simulink model "MyPTControl_RTW"  (Simulink 8.7)
settings: Solver=ode1  SolverMode=SingleTasking  StartTime=0.0  StopTime=inf  FixedStep=0.001  RelTol=1e-3
PreLoadFcn:
  | vehicle = 'Car'; if ~length(which('cmcmd')), cmenv; end
  | MyPTControl_RTW_bus
InitFcn:
  | vehicle = 'Car'; if ~length(which('cmcmd')), cmenv; end
  | MyPTControl_RTW_bus
undefined symbols (not defined in the file or in its folder): EngineOut_Load, EngineOut_set_ISC, Ignition, ISGOut_Load, OperationState
libraries: simulink x11
Description:
  | CarMaker Plug-in Model Target
settings Model: Creator=ml  LastModifiedBy=IPG
settings DataIOCC: SignalLoggingSaveFormat=ModelDataLogs
settings OptimizationCC: ExpressionDepthLimit=2147483647
settings DebuggingCC: FcnCallInpInsideContextMsg=EnableAllAsWarning  StateNameClashWarn=warning
settings HardwareCC: TargetHWDeviceType=32-bit Generic  ProdEqTarget=off
settings RTWCC: SystemTargetFile=CarMaker.tlc  TemplateMakefile=CarMaker_unix-win64.tmf  Description=CarMaker Plug-in Model Target
settings CodeAppCC: MaxIdLength=127
settings STFCustomTargetCC: ModelReferenceCompliant=off  GeneratePreprocessorConditionals=Disable all  MultiInstanceERTCode=on  CodeInterfacePackaging=Reusable function  CPPClassGenCompliant=on  GRTInterface=off  GenerateAllocFcn=on  SystemTargetFile=CarMaker.tlc
settings GRTTargetCC: ModelReferenceCompliant=off  ParMdlRefBuildCompliant=off  CompOptLevelCompliant=off  ConcurrentExecutionCompliant=off  CombineOutputUpdateFcns=off  MatFileLogging=off  MultiInstanceERTCode=on  CodeInterfacePackaging=Reusable function  GenerateAllocFcn=on  UseToolchainInfoCompliant=off
settings CustomProperty: DataType=string  Value=..
settings EnumStrPairs: String=Car

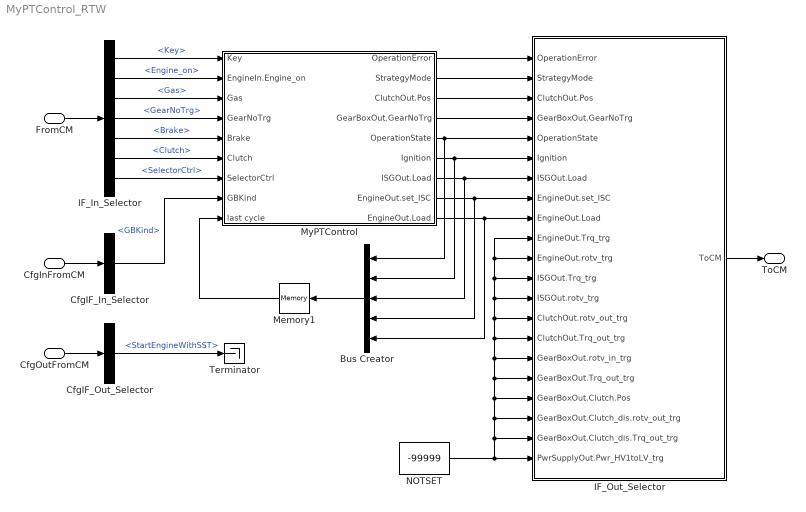
== system MyPTControl_RTW ==
  FromCM : Inport  OutDataTypeStr=Bus: cmPTControlIn
  CfgInFromCM : Inport  Port=2  OutDataTypeStr=Bus: cmPTControlCfgIn
  CfgOutFromCM : Inport  Port=3  OutDataTypeStr=Bus: cmPTControlCfgOut
  Bus Creator : BusCreator  Inputs=5
  CfgIF_In_Selector : BusSelector  OutputSignals=GearBox.GBKind
  CfgIF_Out_Selector : BusSelector  OutputSignals=StartEngineWithSST
  IF_In_Selector : BusSelector  OutputSignals=Key,EngineIn.Engine_on,Gas,GearNoTrg,Brake,Clutch,SelectorCtrl
  IF_Out_Selector : Subsystem  mask(Signal Selection){}
      mask help: Signal Selection Block
      settings: OpenFcn=cmSignalSelect('SignalSelection_CB',gcb)
  Memory1 : Memory
  MyPTControl : Subsystem
  NOTSET : Constant  Value=-99999
  Terminator : Terminator
  ToCM : Outport  OutDataTypeStr=Bus: cmPTControlOut
  wires:
  FromCM/1 -> IF_In_Selector/1
  IF_Out_Selector/1(ToCM) -> ToCM/1
  CfgInFromCM/1 -> CfgIF_In_Selector/1
  CfgOutFromCM/1 -> CfgIF_Out_Selector/1
  Bus Creator/1 -> Memory1/1
  Memory1/1 -> MyPTControl/9(last cycle)
  MyPTControl/5(OperationState) -> Bus Creator/1, IF_Out_Selector/5(OperationState)
  MyPTControl/6(Ignition) -> Bus Creator/2, IF_Out_Selector/6(Ignition)
  MyPTControl/7(ISGOut.Load) -> Bus Creator/3, IF_Out_Selector/7(ISGOut.Load)
  MyPTControl/8(EngineOut.set_ISC) -> Bus Creator/4, IF_Out_Selector/8(EngineOut.set_ISC)
  MyPTControl/9(EngineOut.Load) -> Bus Creator/5, IF_Out_Selector/9(EngineOut.Load)
  MyPTControl/1(OperationError) -> IF_Out_Selector/1(OperationError)
  MyPTControl/2(StrategyMode) -> IF_Out_Selector/2(StrategyMode)
  MyPTControl/3(ClutchOut.Pos) -> IF_Out_Selector/3(ClutchOut.Pos)
  MyPTControl/4(GearBoxOut.GearNoTrg) -> IF_Out_Selector/4(GearBoxOut.GearNoTrg)
  IF_In_Selector/1 -> MyPTControl/1(Key)  "<Key>"
  IF_In_Selector/2 -> MyPTControl/2(EngineIn.Engine_on)  "<Engine_on>"
  IF_In_Selector/3 -> MyPTControl/3(Gas)  "<Gas>"
  IF_In_Selector/4 -> MyPTControl/4(GearNoTrg)  "<GearNoTrg>"
  IF_In_Selector/5 -> MyPTControl/5(Brake)  "<Brake>"
  IF_In_Selector/6 -> MyPTControl/6(Clutch)  "<Clutch>"
  IF_In_Selector/7 -> MyPTControl/7(SelectorCtrl)  "<SelectorCtrl>"
  CfgIF_In_Selector/1 -> MyPTControl/8(GBKind)  "<GBKind>"
  CfgIF_Out_Selector/1 -> Terminator/1  "<StartEngineWithSST>"
  NOTSET/1 -> IF_Out_Selector/21(PwrSupplyOut.Pwr_HV1toLV_trg), IF_Out_Selector/10(EngineOut.Trq_trg), IF_Out_Selector/11(EngineOut.rotv_trg), IF_Out_Selector/12(ISGOut.Trq_trg), IF_Out_Selector/13(ISGOut.rotv_trg), IF_Out_Selector/14(ClutchOut.rotv_out_trg), IF_Out_Selector/15(ClutchOut.Trq_out_trg), IF_Out_Selector/16(GearBoxOut.rotv_in_trg), IF_Out_Selector/17(GearBoxOut.Trq_out_trg), IF_Out_Selector/18(GearBoxOut.Clutch.Pos), IF_Out_Selector/19(GearBoxOut.Clutch_dis.rotv_out_trg), IF_Out_Selector/20(GearBoxOut.Clutch_dis.Trq_out_trg)

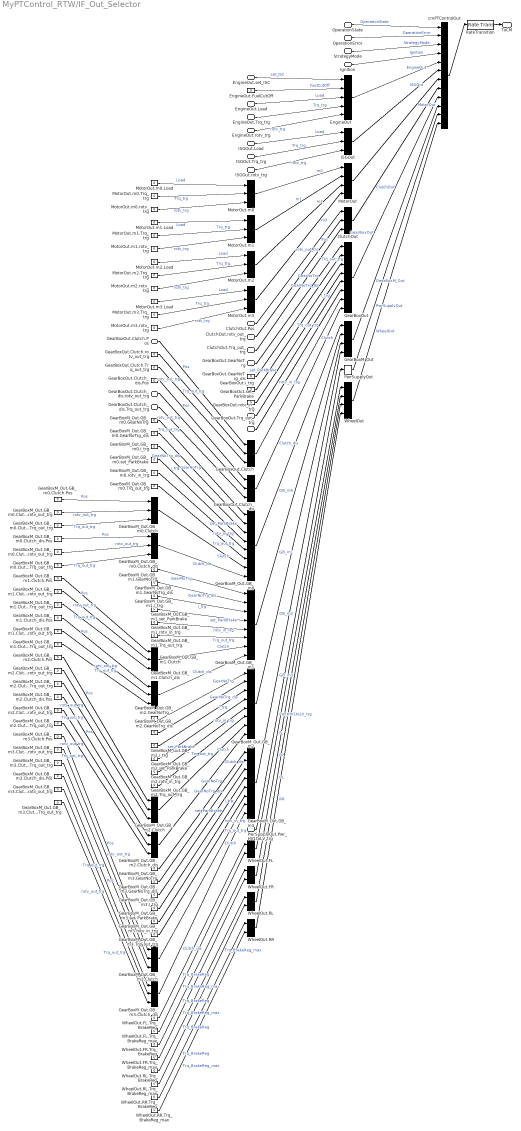
== system MyPTControl_RTW/IF_Out_Selector ==
  OperationError : Inport
  StrategyMode : Inport  Port=2
  ClutchOut.Pos : Inport  Port=3
  GearBoxOut.GearNoTrg : Inport  Port=4
  OperationState : Inport  Port=5
  Ignition : Inport  Port=6
  ISGOut.Load : Inport  Port=7
  EngineOut.set_ISC : Inport  Port=8
  EngineOut.Load : Inport  Port=9
  EngineOut.Trq_trg : Inport  Port=10
  EngineOut.rotv_trg : Inport  Port=11
  ISGOut.Trq_trg : Inport  Port=12
  ISGOut.rotv_trg : Inport  Port=13
  ClutchOut.rotv_out_trg : Inport  Port=14
  ClutchOut.Trq_out_trg : Inport  Port=15
  GearBoxOut.rotv_in_trg : Inport  Port=16
  GearBoxOut.Trq_out_trg : Inport  Port=17
  GearBoxOut.Clutch.Pos : Inport  Port=18
  GearBoxOut.Clutch_dis.rotv_out_trg : Inport  Port=19
  GearBoxOut.Clutch_dis.Trq_out_trg : Inport  Port=20
  PwrSupplyOut.Pwr_HV1toLV_trg : Inport  Port=21
  ClutchOut : BusCreator  Inputs=3
  EngineOut : BusCreator  Inputs=5
  EngineOut.FuelCutOff : Constant  Value=0
  GearBoxM_Out : BusCreator  Inputs=4
  GearBoxM_Out.GB_m{0..3} (4 alike) : BusCreator  Inputs=8
  GearBoxM_Out.GB_m0.Clutch : BusCreator  Inputs=3
  GearBoxM_Out.GB_m0.Clutch.Pos : Constant  Value=0
  GearBoxM_Out.GB_m0.Clutch.Trq_out_trg : Constant  Value=0
  GearBoxM_Out.GB_m0.Clutch.rotv_out_trg : Constant  Value=0
  GearBoxM_Out.GB_m0.Clutch_dis : BusCreator  Inputs=3
  GearBoxM_Out.GB_m0.Clutch_dis.Pos : Constant  Value=0
  GearBoxM_Out.GB_m0.Clutch_dis.Trq_out_trg : Constant  Value=0
  GearBoxM_Out.GB_m0.Clutch_dis.rotv_out_trg : Constant  Value=0
  GearBoxM_Out.GB_m0.GearNoTrg : Constant  Value=0
  GearBoxM_Out.GB_m0.GearNoTrg_dis : Constant  Value=0
  GearBoxM_Out.GB_m0.Trq_out_trg : Constant  Value=0
  GearBoxM_Out.GB_m0.i_trg : Constant  Value=0
  GearBoxM_Out.GB_m0.rotv_in_trg : Constant  Value=0
  GearBoxM_Out.GB_m0.set_ParkBrake : Constant  Value=0
  GearBoxM_Out.GB_m1.Clutch : BusCreator  Inputs=3
  GearBoxM_Out.GB_m1.Clutch.Pos : Constant  Value=0
  GearBoxM_Out.GB_m1.Clutch.Trq_out_trg : Constant  Value=0
  GearBoxM_Out.GB_m1.Clutch.rotv_out_trg : Constant  Value=0
  GearBoxM_Out.GB_m1.Clutch_dis : BusCreator  Inputs=3
  GearBoxM_Out.GB_m1.Clutch_dis.Pos : Constant  Value=0
  GearBoxM_Out.GB_m1.Clutch_dis.Trq_out_trg : Constant  Value=0
  GearBoxM_Out.GB_m1.Clutch_dis.rotv_out_trg : Constant  Value=0
  GearBoxM_Out.GB_m1.GearNoTrg : Constant  Value=0
  GearBoxM_Out.GB_m1.GearNoTrg_dis : Constant  Value=0
  GearBoxM_Out.GB_m1.Trq_out_trg : Constant  Value=0
  GearBoxM_Out.GB_m1.i_trg : Constant  Value=0
  GearBoxM_Out.GB_m1.rotv_in_trg : Constant  Value=0
  GearBoxM_Out.GB_m1.set_ParkBrake : Constant  Value=0
  GearBoxM_Out.GB_m2.Clutch : BusCreator  Inputs=3
  GearBoxM_Out.GB_m2.Clutch.Pos : Constant  Value=0
  GearBoxM_Out.GB_m2.Clutch.Trq_out_trg : Constant  Value=0
  GearBoxM_Out.GB_m2.Clutch.rotv_out_trg : Constant  Value=0
  GearBoxM_Out.GB_m2.Clutch_dis : BusCreator  Inputs=3
  GearBoxM_Out.GB_m2.Clutch_dis.Pos : Constant  Value=0
  GearBoxM_Out.GB_m2.Clutch_dis.Trq_out_trg : Constant  Value=0
  GearBoxM_Out.GB_m2.Clutch_dis.rotv_out_trg : Constant  Value=0
  GearBoxM_Out.GB_m2.GearNoTrg : Constant  Value=0
  GearBoxM_Out.GB_m2.GearNoTrg_dis : Constant  Value=0
  GearBoxM_Out.GB_m2.Trq_out_trg : Constant  Value=0
  GearBoxM_Out.GB_m2.i_trg : Constant  Value=0
  GearBoxM_Out.GB_m2.rotv_in_trg : Constant  Value=0
  GearBoxM_Out.GB_m2.set_ParkBrake : Constant  Value=0
  GearBoxM_Out.GB_m3.Clutch : BusCreator  Inputs=3
  GearBoxM_Out.GB_m3.Clutch.Pos : Constant  Value=0
  GearBoxM_Out.GB_m3.Clutch.Trq_out_trg : Constant  Value=0
  GearBoxM_Out.GB_m3.Clutch.rotv_out_trg : Constant  Value=0
  GearBoxM_Out.GB_m3.Clutch_dis : BusCreator  Inputs=3
  GearBoxM_Out.GB_m3.Clutch_dis.Pos : Constant  Value=0
  GearBoxM_Out.GB_m3.Clutch_dis.Trq_out_trg : Constant  Value=0
  GearBoxM_Out.GB_m3.Clutch_dis.rotv_out_trg : Constant  Value=0
  GearBoxM_Out.GB_m3.GearNoTrg : Constant  Value=0
  GearBoxM_Out.GB_m3.GearNoTrg_dis : Constant  Value=0
  GearBoxM_Out.GB_m3.Trq_out_trg : Constant  Value=0
  GearBoxM_Out.GB_m3.i_trg : Constant  Value=0
  GearBoxM_Out.GB_m3.rotv_in_trg : Constant  Value=0
  GearBoxM_Out.GB_m3.set_ParkBrake : Constant  Value=0
  GearBoxOut : BusCreator  Inputs=8
  GearBoxOut.Clutch : BusCreator  Inputs=3
  GearBoxOut.Clutch.Trq_out_trg : Constant  Value=0
  GearBoxOut.Clutch.rotv_out_trg : Constant  Value=0
  GearBoxOut.Clutch_dis : BusCreator  Inputs=3
  GearBoxOut.Clutch_dis.Pos : Constant  Value=0
  GearBoxOut.GearNoTrg_dis : Constant  Value=0
  GearBoxOut.i_trg : Constant  Value=0
  GearBoxOut.set_ParkBrake : Constant  Value=0
  ISGOut : BusCreator  Inputs=3
  MotorOut : BusCreator  Inputs=4
  MotorOut.m{0..3} (4 alike) : BusCreator  Inputs=3
  MotorOut.m0.Load : Constant  Value=0
  MotorOut.m0.Trq_trg : Constant  Value=0
  MotorOut.m0.rotv_trg : Constant  Value=0
  MotorOut.m1.Load : Constant  Value=0
  MotorOut.m1.Trq_trg : Constant  Value=0
  MotorOut.m1.rotv_trg : Constant  Value=0
  MotorOut.m2.Load : Constant  Value=0
  MotorOut.m2.Trq_trg : Constant  Value=0
  MotorOut.m2.rotv_trg : Constant  Value=0
  MotorOut.m3.Load : Constant  Value=0
  MotorOut.m3.Trq_trg : Constant  Value=0
  MotorOut.m3.rotv_trg : Constant  Value=0
  PwrSupplyOut : BusCreator  Inputs=1
  RateTransition : RateTransition  OutPortSampleTime=str2num(get_param(bdroot,'FixedStep'))
  WheelOut : BusCreator  Inputs=4
  WheelOut.FL : BusCreator  Inputs=2
  WheelOut.FL.Trq_BrakeReg : Constant  Value=0
  WheelOut.FL.Trq_BrakeReg_max : Constant  Value=0
  WheelOut.FR : BusCreator  Inputs=2
  WheelOut.FR.Trq_BrakeReg : Constant  Value=0
  WheelOut.FR.Trq_BrakeReg_max : Constant  Value=0
  WheelOut.RL : BusCreator  Inputs=2
  WheelOut.RL.Trq_BrakeReg : Constant  Value=0
  WheelOut.RL.Trq_BrakeReg_max : Constant  Value=0
  WheelOut.RR : BusCreator  Inputs=2
  WheelOut.RR.Trq_BrakeReg : Constant  Value=0
  WheelOut.RR.Trq_BrakeReg_max : Constant  Value=0
  cmPTControlOut : BusCreator  Inputs=12
  ToCM : Outport
  wires:
  RateTransition/1 -> ToCM/1
  cmPTControlOut/1 -> RateTransition/1
  EngineOut/1 -> cmPTControlOut/5  "EngineOut"
  EngineOut.FuelCutOff/1 -> EngineOut/2  "FuelCutOff"
  ISGOut/1 -> cmPTControlOut/6  "ISGOut"
  MotorOut/1 -> cmPTControlOut/7  "MotorOut"
  MotorOut.m0/1 -> MotorOut/1  "m0"
  MotorOut.m0.Load/1 -> MotorOut.m0/1  "Load"
  MotorOut.m0.Trq_trg/1 -> MotorOut.m0/2  "Trq_trg"
  MotorOut.m0.rotv_trg/1 -> MotorOut.m0/3  "rotv_trg"
  MotorOut.m1/1 -> MotorOut/2  "m1"
  MotorOut.m1.Load/1 -> MotorOut.m1/1  "Load"
  MotorOut.m1.Trq_trg/1 -> MotorOut.m1/2  "Trq_trg"
  MotorOut.m1.rotv_trg/1 -> MotorOut.m1/3  "rotv_trg"
  MotorOut.m2/1 -> MotorOut/3  "m2"
  MotorOut.m2.Load/1 -> MotorOut.m2/1  "Load"
  MotorOut.m2.Trq_trg/1 -> MotorOut.m2/2  "Trq_trg"
  MotorOut.m2.rotv_trg/1 -> MotorOut.m2/3  "rotv_trg"
  MotorOut.m3/1 -> MotorOut/4  "m3"
  MotorOut.m3.Load/1 -> MotorOut.m3/1  "Load"
  MotorOut.m3.Trq_trg/1 -> MotorOut.m3/2  "Trq_trg"
  MotorOut.m3.rotv_trg/1 -> MotorOut.m3/3  "rotv_trg"
  ClutchOut/1 -> cmPTControlOut/8  "ClutchOut"
  GearBoxOut/1 -> cmPTControlOut/9  "GearBoxOut"
  GearBoxOut.GearNoTrg_dis/1 -> GearBoxOut/2  "GearNoTrg_dis"
  GearBoxOut.i_trg/1 -> GearBoxOut/3  "i_trg"
  GearBoxOut.set_ParkBrake/1 -> GearBoxOut/4  "set_ParkBrake"
  GearBoxOut.Clutch/1 -> GearBoxOut/7  "Clutch"
  GearBoxOut.Clutch.rotv_out_trg/1 -> GearBoxOut.Clutch/2  "rotv_out_trg"
  GearBoxOut.Clutch.Trq_out_trg/1 -> GearBoxOut.Clutch/3  "Trq_out_trg"
  GearBoxOut.Clutch_dis/1 -> GearBoxOut/8  "Clutch_dis"
  GearBoxOut.Clutch_dis.Pos/1 -> GearBoxOut.Clutch_dis/1  "Pos"
  GearBoxM_Out/1 -> cmPTControlOut/10  "GearBoxM_Out"
  GearBoxM_Out.GB_m0/1 -> GearBoxM_Out/1  "GB_m0"
  GearBoxM_Out.GB_m0.GearNoTrg/1 -> GearBoxM_Out.GB_m0/1  "GearNoTrg"
  GearBoxM_Out.GB_m0.GearNoTrg_dis/1 -> GearBoxM_Out.GB_m0/2  "GearNoTrg_dis"
  GearBoxM_Out.GB_m0.i_trg/1 -> GearBoxM_Out.GB_m0/3  "i_trg"
  GearBoxM_Out.GB_m0.set_ParkBrake/1 -> GearBoxM_Out.GB_m0/4  "set_ParkBrake"
  GearBoxM_Out.GB_m0.rotv_in_trg/1 -> GearBoxM_Out.GB_m0/5  "rotv_in_trg"
  GearBoxM_Out.GB_m0.Trq_out_trg/1 -> GearBoxM_Out.GB_m0/6  "Trq_out_trg"
  GearBoxM_Out.GB_m0.Clutch/1 -> GearBoxM_Out.GB_m0/7  "Clutch"
  GearBoxM_Out.GB_m0.Clutch.Pos/1 -> GearBoxM_Out.GB_m0.Clutch/1  "Pos"
  GearBoxM_Out.GB_m0.Clutch.rotv_out_trg/1 -> GearBoxM_Out.GB_m0.Clutch/2  "rotv_out_trg"
  GearBoxM_Out.GB_m0.Clutch.Trq_out_trg/1 -> GearBoxM_Out.GB_m0.Clutch/3  "Trq_out_trg"
  GearBoxM_Out.GB_m0.Clutch_dis/1 -> GearBoxM_Out.GB_m0/8  "Clutch_dis"
  GearBoxM_Out.GB_m0.Clutch_dis.Pos/1 -> GearBoxM_Out.GB_m0.Clutch_dis/1  "Pos"
  GearBoxM_Out.GB_m0.Clutch_dis.rotv_out_trg/1 -> GearBoxM_Out.GB_m0.Clutch_dis/2  "rotv_out_trg"
  GearBoxM_Out.GB_m0.Clutch_dis.Trq_out_trg/1 -> GearBoxM_Out.GB_m0.Clutch_dis/3  "Trq_out_trg"
  GearBoxM_Out.GB_m1/1 -> GearBoxM_Out/2  "GB_m1"
  GearBoxM_Out.GB_m1.GearNoTrg/1 -> GearBoxM_Out.GB_m1/1  "GearNoTrg"
  GearBoxM_Out.GB_m1.GearNoTrg_dis/1 -> GearBoxM_Out.GB_m1/2  "GearNoTrg_dis"
  GearBoxM_Out.GB_m1.i_trg/1 -> GearBoxM_Out.GB_m1/3  "i_trg"
  GearBoxM_Out.GB_m1.set_ParkBrake/1 -> GearBoxM_Out.GB_m1/4  "set_ParkBrake"
  GearBoxM_Out.GB_m1.rotv_in_trg/1 -> GearBoxM_Out.GB_m1/5  "rotv_in_trg"
  GearBoxM_Out.GB_m1.Trq_out_trg/1 -> GearBoxM_Out.GB_m1/6  "Trq_out_trg"
  GearBoxM_Out.GB_m1.Clutch/1 -> GearBoxM_Out.GB_m1/7  "Clutch"
  GearBoxM_Out.GB_m1.Clutch.Pos/1 -> GearBoxM_Out.GB_m1.Clutch/1  "Pos"
  GearBoxM_Out.GB_m1.Clutch.rotv_out_trg/1 -> GearBoxM_Out.GB_m1.Clutch/2  "rotv_out_trg"
  GearBoxM_Out.GB_m1.Clutch.Trq_out_trg/1 -> GearBoxM_Out.GB_m1.Clutch/3  "Trq_out_trg"
  GearBoxM_Out.GB_m1.Clutch_dis/1 -> GearBoxM_Out.GB_m1/8  "Clutch_dis"
  GearBoxM_Out.GB_m1.Clutch_dis.Pos/1 -> GearBoxM_Out.GB_m1.Clutch_dis/1  "Pos"
  GearBoxM_Out.GB_m1.Clutch_dis.rotv_out_trg/1 -> GearBoxM_Out.GB_m1.Clutch_dis/2  "rotv_out_trg"
  GearBoxM_Out.GB_m1.Clutch_dis.Trq_out_trg/1 -> GearBoxM_Out.GB_m1.Clutch_dis/3  "Trq_out_trg"
  GearBoxM_Out.GB_m2/1 -> GearBoxM_Out/3  "GB_m2"
  GearBoxM_Out.GB_m2.GearNoTrg/1 -> GearBoxM_Out.GB_m2/1  "GearNoTrg"
  GearBoxM_Out.GB_m2.GearNoTrg_dis/1 -> GearBoxM_Out.GB_m2/2  "GearNoTrg_dis"
  GearBoxM_Out.GB_m2.i_trg/1 -> GearBoxM_Out.GB_m2/3  "i_trg"
  GearBoxM_Out.GB_m2.set_ParkBrake/1 -> GearBoxM_Out.GB_m2/4  "set_ParkBrake"
  GearBoxM_Out.GB_m2.rotv_in_trg/1 -> GearBoxM_Out.GB_m2/5  "rotv_in_trg"
  GearBoxM_Out.GB_m2.Trq_out_trg/1 -> GearBoxM_Out.GB_m2/6  "Trq_out_trg"
  GearBoxM_Out.GB_m2.Clutch/1 -> GearBoxM_Out.GB_m2/7  "Clutch"
  GearBoxM_Out.GB_m2.Clutch.Pos/1 -> GearBoxM_Out.GB_m2.Clutch/1  "Pos"
  GearBoxM_Out.GB_m2.Clutch.rotv_out_trg/1 -> GearBoxM_Out.GB_m2.Clutch/2  "rotv_out_trg"
  GearBoxM_Out.GB_m2.Clutch.Trq_out_trg/1 -> GearBoxM_Out.GB_m2.Clutch/3  "Trq_out_trg"
  GearBoxM_Out.GB_m2.Clutch_dis/1 -> GearBoxM_Out.GB_m2/8  "Clutch_dis"
  GearBoxM_Out.GB_m2.Clutch_dis.Pos/1 -> GearBoxM_Out.GB_m2.Clutch_dis/1  "Pos"
  GearBoxM_Out.GB_m2.Clutch_dis.rotv_out_trg/1 -> GearBoxM_Out.GB_m2.Clutch_dis/2  "rotv_out_trg"
  GearBoxM_Out.GB_m2.Clutch_dis.Trq_out_trg/1 -> GearBoxM_Out.GB_m2.Clutch_dis/3  "Trq_out_trg"
  GearBoxM_Out.GB_m3/1 -> GearBoxM_Out/4  "GB_m3"
  GearBoxM_Out.GB_m3.GearNoTrg/1 -> GearBoxM_Out.GB_m3/1  "GearNoTrg"
  GearBoxM_Out.GB_m3.GearNoTrg_dis/1 -> GearBoxM_Out.GB_m3/2  "GearNoTrg_dis"
  GearBoxM_Out.GB_m3.i_trg/1 -> GearBoxM_Out.GB_m3/3  "i_trg"
  GearBoxM_Out.GB_m3.set_ParkBrake/1 -> GearBoxM_Out.GB_m3/4  "set_ParkBrake"
  GearBoxM_Out.GB_m3.rotv_in_trg/1 -> GearBoxM_Out.GB_m3/5  "rotv_in_trg"
  GearBoxM_Out.GB_m3.Trq_out_trg/1 -> GearBoxM_Out.GB_m3/6  "Trq_out_trg"
  GearBoxM_Out.GB_m3.Clutch/1 -> GearBoxM_Out.GB_m3/7  "Clutch"
  GearBoxM_Out.GB_m3.Clutch.Pos/1 -> GearBoxM_Out.GB_m3.Clutch/1  "Pos"
  GearBoxM_Out.GB_m3.Clutch.rotv_out_trg/1 -> GearBoxM_Out.GB_m3.Clutch/2  "rotv_out_trg"
  GearBoxM_Out.GB_m3.Clutch.Trq_out_trg/1 -> GearBoxM_Out.GB_m3.Clutch/3  "Trq_out_trg"
  GearBoxM_Out.GB_m3.Clutch_dis/1 -> GearBoxM_Out.GB_m3/8  "Clutch_dis"
  GearBoxM_Out.GB_m3.Clutch_dis.Pos/1 -> GearBoxM_Out.GB_m3.Clutch_dis/1  "Pos"
  GearBoxM_Out.GB_m3.Clutch_dis.rotv_out_trg/1 -> GearBoxM_Out.GB_m3.Clutch_dis/2  "rotv_out_trg"
  GearBoxM_Out.GB_m3.Clutch_dis.Trq_out_trg/1 -> GearBoxM_Out.GB_m3.Clutch_dis/3  "Trq_out_trg"
  PwrSupplyOut/1 -> cmPTControlOut/11  "PwrSupplyOut"
  WheelOut/1 -> cmPTControlOut/12  "WheelOut"
  WheelOut.FL/1 -> WheelOut/1  "FL"
  WheelOut.FL.Trq_BrakeReg/1 -> WheelOut.FL/1  "Trq_BrakeReg"
  WheelOut.FL.Trq_BrakeReg_max/1 -> WheelOut.FL/2  "Trq_BrakeReg_max"
  WheelOut.FR/1 -> WheelOut/2  "FR"
  WheelOut.FR.Trq_BrakeReg/1 -> WheelOut.FR/1  "Trq_BrakeReg"
  WheelOut.FR.Trq_BrakeReg_max/1 -> WheelOut.FR/2  "Trq_BrakeReg_max"
  WheelOut.RL/1 -> WheelOut/3  "RL"
  WheelOut.RL.Trq_BrakeReg/1 -> WheelOut.RL/1  "Trq_BrakeReg"
  WheelOut.RL.Trq_BrakeReg_max/1 -> WheelOut.RL/2  "Trq_BrakeReg_max"
  WheelOut.RR/1 -> WheelOut/4  "RR"
  WheelOut.RR.Trq_BrakeReg/1 -> WheelOut.RR/1  "Trq_BrakeReg"
  WheelOut.RR.Trq_BrakeReg_max/1 -> WheelOut.RR/2  "Trq_BrakeReg_max"
  OperationError/1 -> cmPTControlOut/2  "OperationError"
  StrategyMode/1 -> cmPTControlOut/3  "StrategyMode"
  ClutchOut.Pos/1 -> ClutchOut/1  "Pos"
  GearBoxOut.GearNoTrg/1 -> GearBoxOut/1  "GearNoTrg"
  OperationState/1 -> cmPTControlOut/1  "OperationState"
  Ignition/1 -> cmPTControlOut/4  "Ignition"
  ISGOut.Load/1 -> ISGOut/1  "Load"
  EngineOut.set_ISC/1 -> EngineOut/1  "set_ISC"
  EngineOut.Load/1 -> EngineOut/3  "Load"
  EngineOut.Trq_trg/1 -> EngineOut/4  "Trq_trg"
  EngineOut.rotv_trg/1 -> EngineOut/5  "rotv_trg"
  ISGOut.Trq_trg/1 -> ISGOut/2  "Trq_trg"
  ISGOut.rotv_trg/1 -> ISGOut/3  "rotv_trg"
  ClutchOut.rotv_out_trg/1 -> ClutchOut/2  "rotv_out_trg"
  ClutchOut.Trq_out_trg/1 -> ClutchOut/3  "Trq_out_trg"
  GearBoxOut.rotv_in_trg/1 -> GearBoxOut/5  "rotv_in_trg"
  GearBoxOut.Trq_out_trg/1 -> GearBoxOut/6  "Trq_out_trg"
  GearBoxOut.Clutch.Pos/1 -> GearBoxOut.Clutch/1  "Pos"
  GearBoxOut.Clutch_dis.rotv_out_trg/1 -> GearBoxOut.Clutch_dis/2  "rotv_out_trg"
  GearBoxOut.Clutch_dis.Trq_out_trg/1 -> GearBoxOut.Clutch_dis/3  "Trq_out_trg"
  PwrSupplyOut.Pwr_HV1toLV_trg/1 -> PwrSupplyOut/1  "Pwr_HV1toLV_trg"

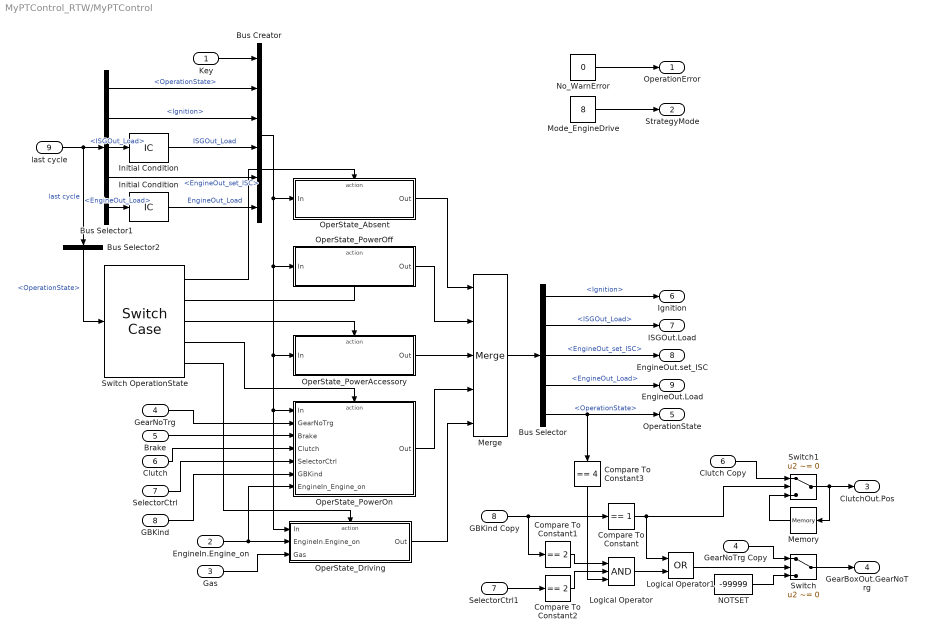
== system MyPTControl_RTW/MyPTControl ==
  Key : Inport
  EngineIn.Engine_on : Inport  Port=2
  Gas : Inport  Port=3
  GearNoTrg : Inport  Port=4
  Brake : Inport  Port=5
  Clutch : Inport  Port=6
  SelectorCtrl : Inport  Port=7
  GBKind : Inport  Port=8
  last cycle : Inport  Port=9
  Bus Creator : BusCreator  Inputs=6
  Bus Selector : BusSelector  OutputSignals=Ignition,ISGOut_Load,EngineOut_set_ISC,EngineOut_Load,OperationState
  Bus Selector1 : BusSelector  OutputSignals=OperationState,Ignition,ISGOut_Load,EngineOut_set_ISC,EngineOut_Load
  Bus Selector2 : BusSelector  OutputSignals=OperationState
  Clutch Copy : InportShadow  Port=6
  Compare To Constant : simulink/Logic and Bit Operations/Compare To Constant  relop===  const=1  OutDataTypeStr=uint8  ZeroCross=off
  Compare To Constant1 : simulink/Logic and Bit Operations/Compare To Constant  relop===  const=2  OutDataTypeStr=uint8  ZeroCross=off
  Compare To Constant2 : simulink/Logic and Bit Operations/Compare To Constant  relop===  const=2  OutDataTypeStr=uint8  ZeroCross=off
  Compare To Constant3 : simulink/Logic and Bit Operations/Compare To Constant  relop===  const=4  OutDataTypeStr=uint8  ZeroCross=off
  GBKind Copy : InportShadow  Port=8
  GearNoTrg Copy : InportShadow  Port=4
  Initial Condition : InitialCondition  Value=0
  "Initial Condition " : InitialCondition  Value=0
  Logical Operator : Logic  Inputs=3  AllPortsSameDT=off  OutDataTypeStr=boolean
  Logical Operator1 : Logic  Operator=OR  AllPortsSameDT=off  OutDataTypeStr=boolean
  Memory : Memory
  Merge : Merge  Inputs=5
  Mode_EngineDrive : Constant  Value=8
  NOTSET : Constant  Value=-99999
  No_WarnError : Constant  Value=0
  OperState_Absent : Subsystem  TreatAsAtomicUnit=on
  OperState_Driving : Subsystem  TreatAsAtomicUnit=on
  OperState_PowerAccessory : Subsystem  TreatAsAtomicUnit=on
  OperState_PowerOff : Subsystem  TreatAsAtomicUnit=on
  OperState_PowerOn : Subsystem  TreatAsAtomicUnit=on
  SelectorCtrl1 : InportShadow  Port=7
  Switch : Switch  Criteria=u2 ~= 0
  Switch OperationState : SwitchCase  CaseConditions={0 1 2 3}
  Switch1 : Switch  Criteria=u2 ~= 0
  OperationError : Outport
  StrategyMode : Outport  Port=2
  ClutchOut.Pos : Outport  Port=3
  GearBoxOut.GearNoTrg : Outport  Port=4
  OperationState : Outport  Port=5
  Ignition : Outport  Port=6
  ISGOut.Load : Outport  Port=7
  EngineOut.set_ISC : Outport  Port=8
  EngineOut.Load : Outport  Port=9
  wires:
  Compare To Constant3/1 -> Logical Operator/3
  GBKind Copy/1 -> Compare To Constant1/1, Compare To Constant/1
  SelectorCtrl1/1 -> Compare To Constant2/1
  OperState_Absent/1(Out) -> Merge/1
  Initial Condition/1 -> Bus Creator/4  "ISGOut_Load"
  "Initial Condition "/1 -> Bus Creator/6  "EngineOut_Load"
  Memory/1 -> Switch1/3
  Clutch Copy/1 -> Switch1/1
  Switch1/1 -> Memory/1, ClutchOut.Pos/1
  Switch/1 -> GearBoxOut.GearNoTrg/1
  GearNoTrg Copy/1 -> Switch/1
  NOTSET/1 -> Switch/3
  Logical Operator1/1 -> Switch/2
  Compare To Constant/1 -> Switch1/2, Logical Operator1/1
  Logical Operator/1 -> Logical Operator1/2
  Compare To Constant2/1 -> Logical Operator/2
  Compare To Constant1/1 -> Logical Operator/1
  Merge/1 -> Bus Selector/1
  OperState_Driving/1(Out) -> Merge/5
  OperState_PowerOn/1(Out) -> Merge/4
  OperState_PowerAccessory/1(Out) -> Merge/3
  OperState_PowerOff/1(Out) -> Merge/2
  Bus Selector1/5 -> "Initial Condition "/1  "<EngineOut_Load>"
  Bus Selector1/4 -> Bus Creator/5  "<EngineOut_set_ISC>"
  Bus Selector1/3 -> Initial Condition/1  "<ISGOut_Load>"
  Bus Selector1/2 -> Bus Creator/3  "<Ignition>"
  Bus Selector1/1 -> Bus Creator/2  "<OperationState>"
  Switch OperationState/1 -> OperState_Absent/Action
  Switch OperationState/5 -> OperState_Driving/Action
  Switch OperationState/4 -> OperState_PowerOn/Action
  Switch OperationState/2 -> OperState_PowerOff/Action
  Gas/1 -> OperState_Driving/3(Gas)
  GBKind/1 -> OperState_PowerOn/6(GBKind)
  SelectorCtrl/1 -> OperState_PowerOn/5(SelectorCtrl)
  Clutch/1 -> OperState_PowerOn/4(Clutch)
  Brake/1 -> OperState_PowerOn/3(Brake)
  GearNoTrg/1 -> OperState_PowerOn/2(GearNoTrg)
  Bus Selector/4 -> EngineOut.Load/1  "<EngineOut_Load>"
  Bus Selector/3 -> EngineOut.set_ISC/1  "<EngineOut_set_ISC>"
  Bus Selector/2 -> ISGOut.Load/1  "<ISGOut_Load>"
  Bus Creator/1 -> OperState_Driving/1(In), OperState_PowerOn/1(In), OperState_PowerAccessory/1(In), OperState_PowerOff/1(In), OperState_Absent/1(In)
  Key/1 -> Bus Creator/1
  Bus Selector2/1 -> Switch OperationState/1  "<OperationState>"
  last cycle/1 -> Bus Selector1/1, Bus Selector2/1  "last cycle"
  EngineIn.Engine_on/1 -> OperState_Driving/2(EngineIn.Engine_on), OperState_PowerOn/7(EngineIn_Engine_on)
  Bus Selector/5 -> Compare To Constant3/1, OperationState/1  "<OperationState>"
  Bus Selector/1 -> Ignition/1  "<Ignition>"
  Switch OperationState/3 -> OperState_PowerAccessory/Action
  Mode_EngineDrive/1 -> StrategyMode/1
  No_WarnError/1 -> OperationError/1

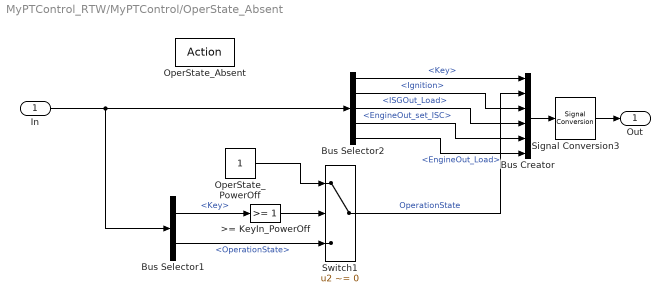
== system MyPTControl_RTW/MyPTControl/OperState_Absent ==
  In : Inport
  OperState_Absent : ActionPort  ActionType=case
  >= KeyIn_PowerOff : simulink/Logic and Bit Operations/Compare To Constant  relop=>=  const=1  OutDataTypeStr=uint8  ZeroCross=off
  Bus Creator : BusCreator  Inputs=6
  Bus Selector1 : BusSelector  OutputSignals=Key,OperationState
  Bus Selector2 : BusSelector  OutputSignals=Key,Ignition,ISGOut_Load,EngineOut_set_ISC,EngineOut_Load
  OperState_PowerOff : Constant
  Signal Conversion3 : SignalConversion  ConversionOutput=Bus copy  OverrideOpt=off
  Switch1 : Switch  Criteria=u2 ~= 0  Threshold=1
  Out : Outport
  wires:
  >= KeyIn_PowerOff/1 -> Switch1/2
  Bus Selector2/5 -> Bus Creator/6  "<EngineOut_Load>"
  Bus Selector2/4 -> Bus Creator/5  "<EngineOut_set_ISC>"
  Bus Selector2/3 -> Bus Creator/4  "<ISGOut_Load>"
  Bus Selector2/2 -> Bus Creator/3  "<Ignition>"
  Bus Selector2/1 -> Bus Creator/1  "<Key>"
  Switch1/1 -> Bus Creator/2  "OperationState"
  Signal Conversion3/1 -> Out/1
  Bus Creator/1 -> Signal Conversion3/1
  Bus Selector1/2 -> Switch1/3  "<OperationState>"
  OperState_PowerOff/1 -> Switch1/1
  Bus Selector1/1 -> >= KeyIn_PowerOff/1  "<Key>"
  In/1 -> Bus Selector2/1, Bus Selector1/1

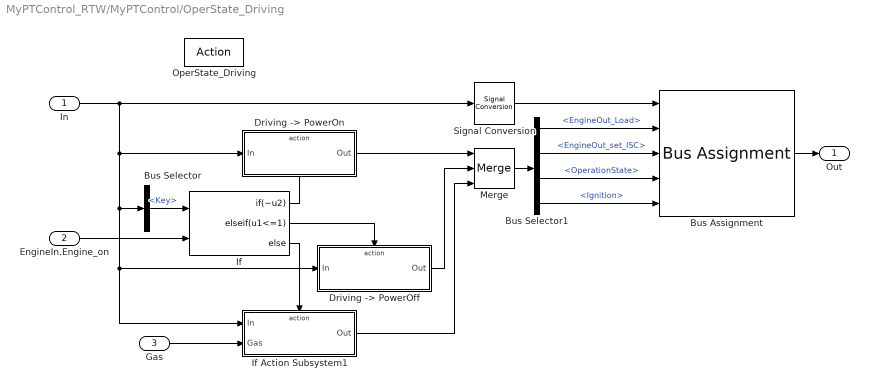
== system MyPTControl_RTW/MyPTControl/OperState_Driving ==
  In : Inport
  EngineIn.Engine_on : Inport  Port=2
  Gas : Inport  Port=3
  OperState_Driving : ActionPort  ActionType=default
  Bus Assignment : BusAssignment  AssignedSignals=EngineOut_Load,EngineOut_set_ISC,OperationState,Ignition
  Bus Selector : BusSelector  OutputSignals=Key
  Bus Selector1 : BusSelector  OutputSignals=EngineOut_Load,EngineOut_set_ISC,OperationState,Ignition
  "Driving -> PowerOff" : Subsystem  TreatAsAtomicUnit=on
  "Driving -> PowerOn" : Subsystem  TreatAsAtomicUnit=on
  If : If  NumInputs=2  IfExpression=~u2  ElseIfExpressions=u1<=1
  If Action Subsystem1 : Subsystem  TreatAsAtomicUnit=on
  Merge : Merge  Inputs=3
  Signal Conversion : SignalConversion  ConversionOutput=Bus copy  OverrideOpt=off
  Out : Outport
  wires:
  Signal Conversion/1 -> Bus Assignment/1
  "Driving -> PowerOff"/1(Out) -> Merge/2
  Gas/1 -> If Action Subsystem1/2(Gas)
  Bus Selector1/4 -> Bus Assignment/5  "<Ignition>"
  Bus Selector1/3 -> Bus Assignment/4  "<OperationState>"
  Bus Selector1/2 -> Bus Assignment/3  "<EngineOut_set_ISC>"
  Bus Selector1/1 -> Bus Assignment/2  "<EngineOut_Load>"
  "Driving -> PowerOn"/1(Out) -> Merge/1
  If Action Subsystem1/1(Out) -> Merge/3
  EngineIn.Engine_on/1 -> If/2
  Bus Selector/1 -> If/1  "<Key>"
  If/2 -> "Driving -> PowerOff"/Action
  If/1 -> "Driving -> PowerOn"/Action
  If/3 -> If Action Subsystem1/Action
  In/1 -> Signal Conversion/1, If Action Subsystem1/1(In), "Driving -> PowerOff"/1(In), Bus Selector/1, "Driving -> PowerOn"/1(In)
  Bus Assignment/1 -> Out/1
  Merge/1 -> Bus Selector1/1

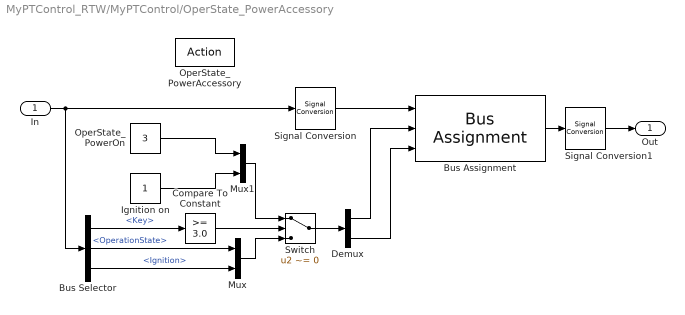
== system MyPTControl_RTW/MyPTControl/OperState_PowerAccessory ==
  In : Inport
  OperState_PowerAccessory : ActionPort  ActionType=case
  Bus Assignment : BusAssignment  AssignedSignals=OperationState,Ignition
  Bus Selector : BusSelector  OutputSignals=Key,OperationState,Ignition
  Compare To Constant : simulink/Logic and Bit Operations/Compare To Constant  relop=>=  const=3.0  OutDataTypeStr=uint8  ZeroCross=off
  Demux : Demux  Outputs=2
  Ignition on : Constant
  Mux : Mux  Inputs=2
  Mux1 : Mux  Inputs=2
  OperState_PowerOn : Constant  Value=3
  Signal Conversion : SignalConversion  ConversionOutput=Bus copy  OverrideOpt=off
  Signal Conversion1 : SignalConversion  ConversionOutput=Bus copy  OverrideOpt=off
  Switch : Switch  Criteria=u2 ~= 0  Threshold=3
  Out : Outport
  wires:
  Compare To Constant/1 -> Switch/2
  Signal Conversion1/1 -> Out/1
  Signal Conversion/1 -> Bus Assignment/1
  OperState_PowerOn/1 -> Mux1/1
  In/1 -> Signal Conversion/1, Bus Selector/1
  Bus Assignment/1 -> Signal Conversion1/1
  Ignition on/1 -> Mux1/2
  Mux1/1 -> Switch/1
  Mux/1 -> Switch/3
  Bus Selector/3 -> Mux/2  "<Ignition>"
  Bus Selector/2 -> Mux/1  "<OperationState>"
  Demux/2 -> Bus Assignment/3
  Demux/1 -> Bus Assignment/2
  Switch/1 -> Demux/1
  Bus Selector/1 -> Compare To Constant/1  "<Key>"

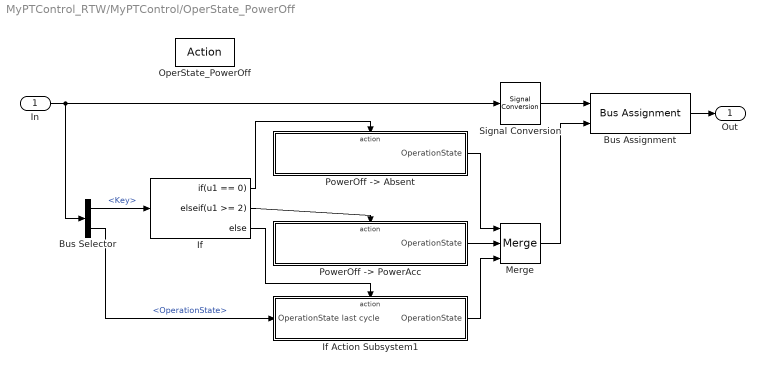
== system MyPTControl_RTW/MyPTControl/OperState_PowerOff ==
  In : Inport
  OperState_PowerOff : ActionPort  ActionType=case
  Bus Assignment : BusAssignment  AssignedSignals=OperationState
  Bus Selector : BusSelector  OutputSignals=Key,OperationState
  If : If  IfExpression=u1 == 0  ElseIfExpressions=u1 >= 2
  If Action Subsystem1 : Subsystem  TreatAsAtomicUnit=on
  Merge : Merge  Inputs=3
  "PowerOff -> Absent" : Subsystem  TreatAsAtomicUnit=on
  "PowerOff -> PowerAcc" : Subsystem  TreatAsAtomicUnit=on
  Signal Conversion : SignalConversion  ConversionOutput=Bus copy  OverrideOpt=off
  Out : Outport
  wires:
  Signal Conversion/1 -> Bus Assignment/1
  Bus Selector/1 -> If/1  "<Key>"
  In/1 -> Signal Conversion/1, Bus Selector/1
  Bus Assignment/1 -> Out/1
  If/3 -> If Action Subsystem1/Action
  If Action Subsystem1/1(OperationState) -> Merge/3
  "PowerOff -> PowerAcc"/1(OperationState) -> Merge/2
  If/2 -> "PowerOff -> PowerAcc"/Action
  Bus Selector/2 -> If Action Subsystem1/1(OperationState last cycle)  "<OperationState>"
  "PowerOff -> Absent"/1(OperationState) -> Merge/1
  Merge/1 -> Bus Assignment/2
  If/1 -> "PowerOff -> Absent"/Action

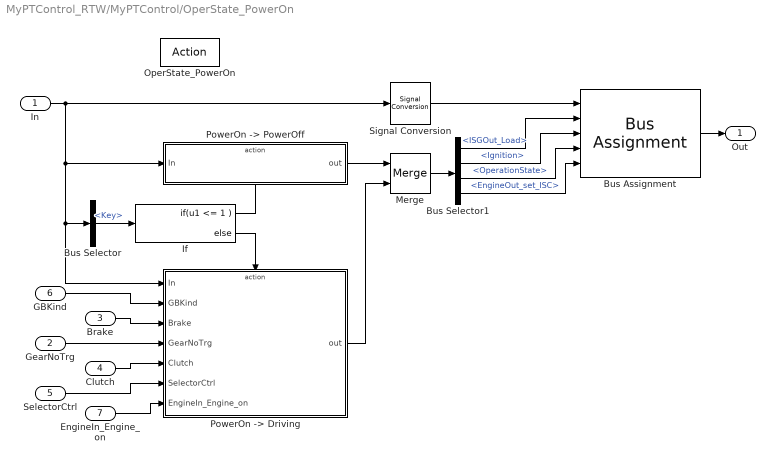
== system MyPTControl_RTW/MyPTControl/OperState_PowerOn ==
  In : Inport
  GearNoTrg : Inport  Port=2
  Brake : Inport  Port=3
  Clutch : Inport  Port=4
  SelectorCtrl : Inport  Port=5
  GBKind : Inport  Port=6
  EngineIn_Engine_on : Inport  Port=7
  OperState_PowerOn : ActionPort  ActionType=case
  Bus Assignment : BusAssignment  AssignedSignals=ISGOut_Load,Ignition,OperationState,EngineOut_set_ISC
  Bus Selector : BusSelector  OutputSignals=Key
  Bus Selector1 : BusSelector  OutputSignals=ISGOut_Load,Ignition,OperationState,EngineOut_set_ISC
  If : If  IfExpression=u1 <= 1
  Merge : Merge
  "PowerOn -> Driving" : Subsystem  TreatAsAtomicUnit=on
  "PowerOn -> PowerOff" : Subsystem  TreatAsAtomicUnit=on
  Signal Conversion : SignalConversion  ConversionOutput=Bus copy  OverrideOpt=off
  Out : Outport
  wires:
  Bus Selector1/4 -> Bus Assignment/5  "<EngineOut_set_ISC>"
  Signal Conversion/1 -> Bus Assignment/1
  "PowerOn -> PowerOff"/1(out) -> Merge/1
  SelectorCtrl/1 -> "PowerOn -> Driving"/6(SelectorCtrl)
  Clutch/1 -> "PowerOn -> Driving"/5(Clutch)
  EngineIn_Engine_on/1 -> "PowerOn -> Driving"/7(EngineIn_Engine_on)
  Bus Selector1/3 -> Bus Assignment/4  "<OperationState>"
  Bus Selector1/2 -> Bus Assignment/3  "<Ignition>"
  Bus Selector1/1 -> Bus Assignment/2  "<ISGOut_Load>"
  GearNoTrg/1 -> "PowerOn -> Driving"/4(GearNoTrg)
  Brake/1 -> "PowerOn -> Driving"/3(Brake)
  GBKind/1 -> "PowerOn -> Driving"/2(GBKind)
  Merge/1 -> Bus Selector1/1
  "PowerOn -> Driving"/1(out) -> Merge/2
  Bus Selector/1 -> If/1  "<Key>"
  Bus Assignment/1 -> Out/1
  In/1 -> Signal Conversion/1, "PowerOn -> PowerOff"/1(In), "PowerOn -> Driving"/1(In), Bus Selector/1
  If/2 -> "PowerOn -> Driving"/Action
  If/1 -> "PowerOn -> PowerOff"/Action

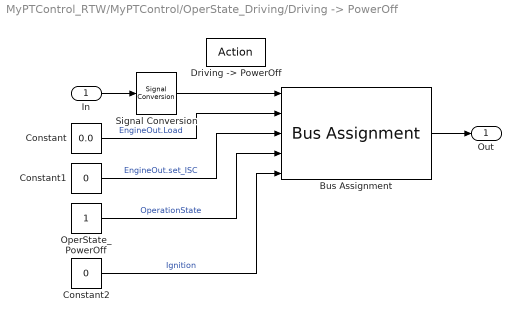
== system MyPTControl_RTW/MyPTControl/OperState_Driving/Driving -> PowerOff ==
  In : Inport
  "Driving -> PowerOff" : ActionPort  ActionType=elseif
  Bus Assignment : BusAssignment  AssignedSignals=EngineOut_Load,EngineOut_set_ISC,Ignition,OperationState
  Constant : Constant  Value=0.0
  Constant1 : Constant  Value=0
  Constant2 : Constant  Value=0
  OperState_PowerOff : Constant
  Signal Conversion : SignalConversion  ConversionOutput=Bus copy  OverrideOpt=off
  Out : Outport  InitialOutput=[0, 0, 0, 0, 0, 0]
  wires:
  Signal Conversion/1 -> Bus Assignment/1
  Constant2/1 -> Bus Assignment/5  "Ignition"
  Constant/1 -> Bus Assignment/2  "EngineOut.Load"
  Bus Assignment/1 -> Out/1
  In/1 -> Signal Conversion/1
  OperState_PowerOff/1 -> Bus Assignment/4  "OperationState"
  Constant1/1 -> Bus Assignment/3  "EngineOut.set_ISC"

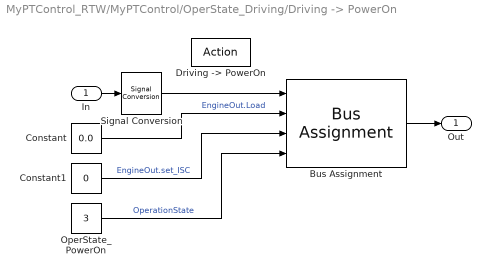
== system MyPTControl_RTW/MyPTControl/OperState_Driving/Driving -> PowerOn ==
  In : Inport
  "Driving -> PowerOn" : ActionPort  ActionType=then
  Bus Assignment : BusAssignment  AssignedSignals=EngineOut_Load,EngineOut_set_ISC,OperationState
  Constant : Constant  Value=0.0
  Constant1 : Constant  Value=0
  OperState_PowerOn : Constant  Value=3
  Signal Conversion : SignalConversion  ConversionOutput=Bus copy  OverrideOpt=off
  Out : Outport  InitialOutput=[0, 0, 0, 0, 0, 0]
  wires:
  Signal Conversion/1 -> Bus Assignment/1
  Bus Assignment/1 -> Out/1
  In/1 -> Signal Conversion/1
  OperState_PowerOn/1 -> Bus Assignment/4  "OperationState"
  Constant1/1 -> Bus Assignment/3  "EngineOut.set_ISC"
  Constant/1 -> Bus Assignment/2  "EngineOut.Load"

== system MyPTControl_RTW/MyPTControl/OperState_Driving/If Action Subsystem1 ==
  In : Inport
  Gas : Inport  Port=2
  Action Port : ActionPort  ActionType=else
  Bus Assignment : BusAssignment  AssignedSignals=EngineOut_Load
  Gain1 : Gain
  Signal Conversion : SignalConversion  ConversionOutput=Bus copy  OverrideOpt=off
  Out : Outport
  wires:
  Signal Conversion/1 -> Bus Assignment/1
  Gain1/1 -> Bus Assignment/2  "EngineOut.Load"
  Bus Assignment/1 -> Out/1
  In/1 -> Signal Conversion/1
  Gas/1 -> Gain1/1

== system MyPTControl_RTW/MyPTControl/OperState_PowerOff/If Action Subsystem1 ==
  OperationState last cycle : Inport
  Action Port : ActionPort  ActionType=else
  OperationState : Outport
  wires:
  OperationState last cycle/1 -> OperationState/1

== system MyPTControl_RTW/MyPTControl/OperState_PowerOff/PowerOff -> Absent ==
  "PowerOff -> Absent" : ActionPort  ActionType=then
  OperState_Absent : Constant  Value=0
  OperationState : Outport  InitialOutput=0
  wires:
  OperState_Absent/1 -> OperationState/1

== system MyPTControl_RTW/MyPTControl/OperState_PowerOff/PowerOff -> PowerAcc ==
  "PowerOff -> PowerAcc" : ActionPort  ActionType=elseif
  OperState_PowerAccesory : Constant  Value=2
  OperationState : Outport  InitialOutput=2
  wires:
  OperState_PowerAccesory/1 -> OperationState/1

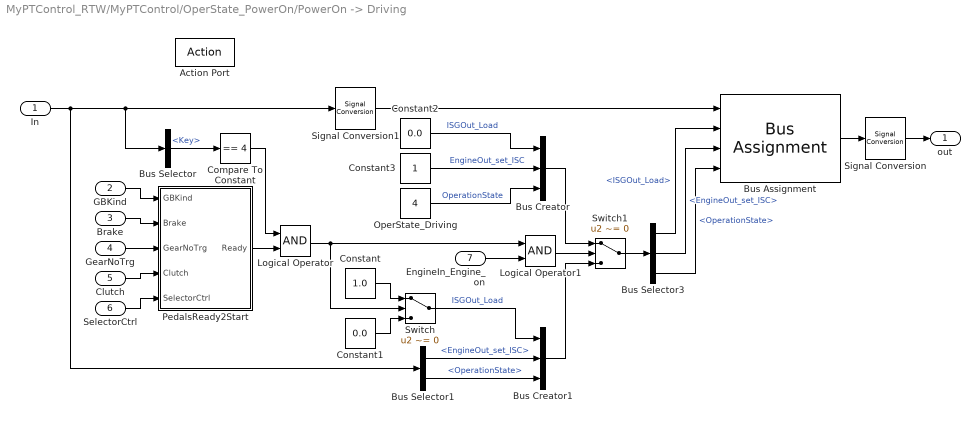
== system MyPTControl_RTW/MyPTControl/OperState_PowerOn/PowerOn -> Driving ==
  In : Inport
  GBKind : Inport  Port=2
  Brake : Inport  Port=3
  GearNoTrg : Inport  Port=4
  Clutch : Inport  Port=5
  SelectorCtrl : Inport  Port=6
  EngineIn_Engine_on : Inport  Port=7
  Action Port : ActionPort  ActionType=else
  Bus Assignment : BusAssignment  AssignedSignals=ISGOut_Load,EngineOut_set_ISC,OperationState
  Bus Creator : BusCreator  Inputs=3
  Bus Creator1 : BusCreator  Inputs=3
  Bus Selector : BusSelector  OutputSignals=Key
  Bus Selector1 : BusSelector  OutputSignals=EngineOut_set_ISC,OperationState
  Bus Selector3 : BusSelector  OutputSignals=ISGOut_Load,EngineOut_set_ISC,OperationState
  Compare To Constant : simulink/Logic and Bit Operations/Compare To Constant  relop===  const=4  OutDataTypeStr=uint8  ZeroCross=off
  Constant : Constant  Value=1.0
  Constant1 : Constant  Value=0.0
  Constant2 : Constant  Value=0.0
  Constant3 : Constant
  Logical Operator : Logic  AllPortsSameDT=off  OutDataTypeStr=boolean
  Logical Operator1 : Logic  AllPortsSameDT=off  OutDataTypeStr=boolean
  OperState_Driving : Constant  Value=4
  PedalsReady2Start : Subsystem
  Signal Conversion : SignalConversion  ConversionOutput=Bus copy  OverrideOpt=off
  Signal Conversion1 : SignalConversion  ConversionOutput=Bus copy  OverrideOpt=off
  Switch : Switch  Criteria=u2 ~= 0
  Switch1 : Switch  Criteria=u2 ~= 0
  out : Outport
  wires:
  Signal Conversion/1 -> out/1
  Bus Selector3/3 -> Bus Assignment/4  "<OperationState>"
  Bus Selector3/2 -> Bus Assignment/3  "<EngineOut_set_ISC>"
  Bus Selector3/1 -> Bus Assignment/2  "<ISGOut_Load>"
  Signal Conversion1/1 -> Bus Assignment/1
  Bus Assignment/1 -> Signal Conversion/1
  Constant3/1 -> Bus Creator/2  "EngineOut_set_ISC"
  Constant2/1 -> Bus Creator/1  "ISGOut_Load"
  OperState_Driving/1 -> Bus Creator/3  "OperationState"
  Bus Creator/1 -> Switch1/1
  Switch/1 -> Bus Creator1/1  "ISGOut_Load"
  Switch1/1 -> Bus Selector3/1
  Logical Operator1/1 -> Switch1/2
  Bus Creator1/1 -> Switch1/3
  Bus Selector1/2 -> Bus Creator1/3  "<OperationState>"
  Bus Selector1/1 -> Bus Creator1/2  "<EngineOut_set_ISC>"
  EngineIn_Engine_on/1 -> Logical Operator1/2
  Constant1/1 -> Switch/3
  Constant/1 -> Switch/1
  Logical Operator/1 -> Logical Operator1/1, Switch/2
  SelectorCtrl/1 -> PedalsReady2Start/5(SelectorCtrl)
  Clutch/1 -> PedalsReady2Start/4(Clutch)
  GearNoTrg/1 -> PedalsReady2Start/3(GearNoTrg)
  Brake/1 -> PedalsReady2Start/2(Brake)
  GBKind/1 -> PedalsReady2Start/1(GBKind)
  PedalsReady2Start/1(Ready) -> Logical Operator/2
  Compare To Constant/1 -> Logical Operator/1
  Bus Selector/1 -> Compare To Constant/1  "<Key>"
  In/1 -> Signal Conversion1/1, Bus Selector/1, Bus Selector1/1

== system MyPTControl_RTW/MyPTControl/OperState_PowerOn/PowerOn -> PowerOff ==
  In : Inport
  "PowerOn -> PowerOff" : ActionPort  ActionType=then
  Bus Assignment : BusAssignment  AssignedSignals=ISGOut_Load,Ignition,OperationState
  Constant : Constant  Value=0.0
  Constant1 : Constant  Value=0
  OperState_PowerOff : Constant
  Signal Conversion : SignalConversion  ConversionOutput=Bus copy  OverrideOpt=off
  out : Outport  InitialOutput=[0, 0, 0, 0, 0, 0]
  wires:
  Signal Conversion/1 -> Bus Assignment/1
  Bus Assignment/1 -> out/1
  In/1 -> Signal Conversion/1
  Constant1/1 -> Bus Assignment/3  "Ignition"
  Constant/1 -> Bus Assignment/2  "ISGOut_Load"
  OperState_PowerOff/1 -> Bus Assignment/4  "OperationState"

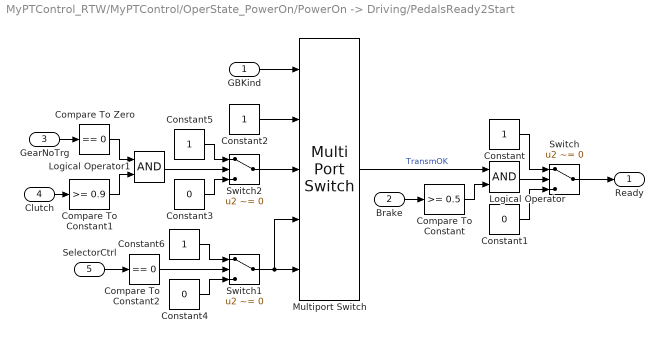
== system MyPTControl_RTW/MyPTControl/OperState_PowerOn/PowerOn -> Driving/PedalsReady2Start ==
  GBKind : Inport
  Brake : Inport  Port=2
  GearNoTrg : Inport  Port=3
  Clutch : Inport  Port=4
  SelectorCtrl : Inport  Port=5
  Compare To Constant : simulink/Logic and Bit Operations/Compare To Constant  relop=>=  const=0.5  OutDataTypeStr=uint8  ZeroCross=off
  Compare To Constant1 : simulink/Logic and Bit Operations/Compare To Constant  relop=>=  const=0.9  OutDataTypeStr=uint8  ZeroCross=off
  Compare To Constant2 : simulink/Logic and Bit Operations/Compare To Constant  relop===  const=0  OutDataTypeStr=uint8  ZeroCross=off
  Compare To Zero : simulink/Logic and Bit Operations/Compare To Zero  relop===  OutDataTypeStr=uint8  ZeroCross=off
  Constant{,2,5..6} (4 alike) : Constant
  Constant1 : Constant  Value=0
  Constant3 : Constant  Value=0
  Constant4 : Constant  Value=0
  Logical Operator : Logic  AllPortsSameDT=off  OutDataTypeStr=boolean
  Logical Operator1 : Logic  AllPortsSameDT=off  OutDataTypeStr=boolean
  Multiport Switch : MultiPortSwitch  DataPortOrder=Zero-based contiguous  Inputs=4  zeroidx=on
  Switch : Switch  Criteria=u2 ~= 0
  Switch1 : Switch  Criteria=u2 ~= 0
  Switch2 : Switch  Criteria=u2 ~= 0
  Ready : Outport
  wires:
  Compare To Constant2/1 -> Switch1/2
  SelectorCtrl/1 -> Compare To Constant2/1
  Compare To Constant1/1 -> Logical Operator1/2
  Compare To Zero/1 -> Logical Operator1/1
  GearNoTrg/1 -> Compare To Zero/1
  Clutch/1 -> Compare To Constant1/1
  Logical Operator1/1 -> Switch2/2
  Constant6/1 -> Switch1/1
  Constant5/1 -> Switch2/1
  Constant4/1 -> Switch1/3
  Constant3/1 -> Switch2/3
  Switch2/1 -> Multiport Switch/3
  Switch1/1 -> Multiport Switch/4, Multiport Switch/5
  Constant2/1 -> Multiport Switch/2
  Constant/1 -> Switch/1
  Constant1/1 -> Switch/3
  Logical Operator/1 -> Switch/2
  Switch/1 -> Ready/1
  Compare To Constant/1 -> Logical Operator/2
  Brake/1 -> Compare To Constant/1
  Multiport Switch/1 -> Logical Operator/1  "TransmOK"
  GBKind/1 -> Multiport Switch/1
